simulink model "motor_model"  (R2023b)
settings: Solver=VariableStepAuto  StartTime=0.0  StopTime=130  RelTol=1e-3
values from neighbouring files (symbols this model uses):
  b = 0.016*2.5    (= 0.04)    [torque.m]
  Im = 0.0059*10    (= 0.059)    [torque.m]
  k = kt    (= 1.45433391507)    [torque.m]
  L = 0.0472    [torque.m]
  R = 2.0    (= 2)    [torque.m]
  Ts = 0.005    [torque.m]
libraries: eeStairGenerator x1
settings Model: Creator=david  LastModifiedBy=david

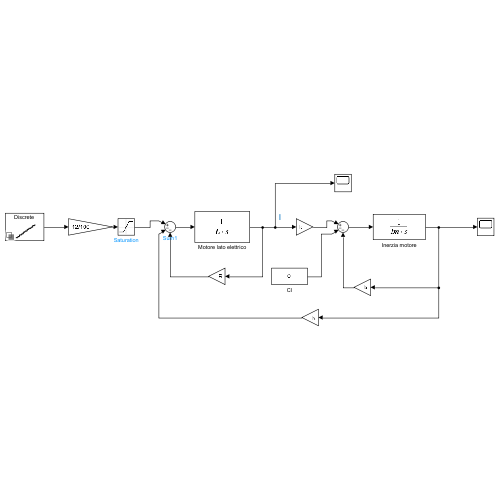
[thumbnail: Simulink's stored preview of the top-level diagram]
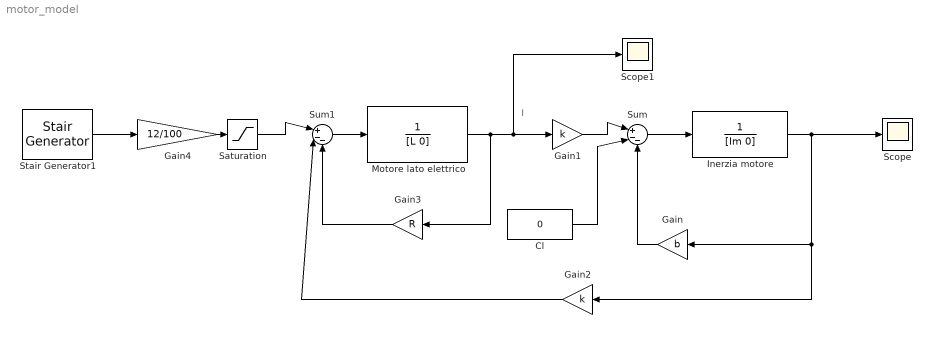
== system motor_model ==
  note: I
  Cl : Constant  Value=0
  Gain : Gain  Gain=b
  Gain1 : Gain  Gain=k
  Gain2 : Gain  Gain=k
  Gain3 : Gain  Gain=R
  Gain4 : Gain  Gain=12/100
  Inerzia motore : TransferFcn  Denominator=[Im 0]
  Motore lato elettrico : TransferFcn  Denominator=[L 0]
  Saturation : Saturate  UpperLimit=12  LowerLimit=0
  Scope : Scope
  Scope1 : Scope
  Stair Generator1 : eeStairGenerator/Stair Generator  LabelModeActiveChoice=Discrete  TimeInput=[0 10 20 30 40 50 60 70 80 90 100]  AmplitudeInput=[0 10 20 30 40 50 60 70 80 90 100]  SampleTime=Ts  RepeatPattern=off  OutDataTypeStr=double
      settings: LibrarySourceBlock=ee_sl_lib/General Control/Stair Generator
  Sum : Sum  Inputs=|+--
  Sum1 : Sum  Inputs=|+--
  wires:
  Motore lato elettrico/1 -> Gain3/1, Scope1/1, Gain1/1
  Gain1/1 -> Sum/1
  Sum/1 -> Inerzia motore/1
  Gain/1 -> Sum/3
  Inerzia motore/1 -> Scope/1, Gain2/1, Gain/1
  Cl/1 -> Sum/2
  Sum1/1 -> Motore lato elettrico/1
  Gain2/1 -> Sum1/2
  Stair Generator1/1 -> Gain4/1
  Saturation/1 -> Sum1/1
  Gain3/1 -> Sum1/3
  Gain4/1 -> Saturation/1
